simulink model "Full_Model_D_R5"  (R2013a)
settings: Solver=ode45  StartTime=0.0  StopTime=sim_length  MaxStep=1e-4  RelTol=1e-3
values from neighbouring files (symbols this model uses):
  A_Height_d = [1  0.03  0.00658443308606; 0  1  0.409781323477; 0  0  0.651439057531]    [Height_Controller_SS_D_Data.mat]    (also in Height_Controller_SS_D_Data[Conflict].mat; Height_Controller_Sample_Time.m = A_d; State_Space_Height_D_1.m = A_d)
  A_Roll_d = [1  0.03  0.0205960284122; 0  1  1.28179110803; 0  0  0.651439057531]    [Roll_Controller_SS_D_Data.mat]    (also in Roll_Controller_SS_D_Data[Conflict].mat; Roll_Controller_Sample_Time.m = A_d; State_Space_Roll_D_1.m = A_d)
  A_Yaw_d = A_d    [State_Space_Yaw_D_2.m]    (also in Yaw_Controller_SS_D_Data.mat = [1  0.03  0.0015367929619; 0  1  0.0956421070134; 0  0  0.65; Yaw_Controller_SS_D_Data[Conflict].mat = [1  0.03  0.0015367929619; 0  1  0.0956421070134; 0  0  0.65)
  B = [0 ... (first row only)    [Height_Controller_Sample_Time.m]    (also in Roll_Controller_Sample_Time.m; State_Space_Height_D_1.m; State_Space_Roll_D_1.m; State_Space_Yaw_D_2.m)
  B_Height_d = [0.000973236713115 0.0940633298008 0.348560942469]    [Height_Controller_SS_D_Data.mat]    (also in Height_Controller_SS_D_Data[Conflict].mat; Height_Controller_Sample_Time.m = B_d; State_Space_Height_D_1.m = B_d)
  B_Roll_d = [0.00304427286801 0.294228977317 0.348560942469]    [Roll_Controller_SS_D_Data.mat]    (also in Roll_Controller_SS_D_Data[Conflict].mat; Roll_Controller_Sample_Time.m = B_d; State_Space_Roll_D_1.m = B_d)
  B_Yaw_d = B_d    [State_Space_Yaw_D_2.m]    (also in Yaw_Controller_SS_D_Data.mat = [0.000231505127222 0.0222444322616 0.348560942469]; Yaw_Controller_SS_D_Data[Conflict].mat = [0.000231505127222 0.0222444322616 0.348560942469])
  C_Height_d = [1 0 0]    [Height_Controller_SS_D_Data.mat]    (also in Height_Controller_SS_D_Data[Conflict].mat; Height_Controller_Sample_Time.m = C_d; State_Space_Height_D_1.m = C_d)
  C_Roll_d = [1  0  0; 0  1  0]    [Roll_Controller_SS_D_Data.mat]    (also in Roll_Controller_SS_D_Data[Conflict].mat; Roll_Controller_Sample_Time.m = C_d; State_Space_Roll_D_1.m = C_d)
  C_Yaw_d = C_d    [State_Space_Yaw_D_2.m]    (also in Yaw_Controller_SS_D_Data.mat = [1  0  0; 0  1  0]; Yaw_Controller_SS_D_Data[Conflict].mat = [1  0  0; 0  1  0])
  Drag = D    [State_Space_Yaw_D_2.m]
  Feed_Forward_Height_d = 2    [Height_Controller_SS_D_Data.mat]    (also in Height_Controller_SS_D_Data[Conflict].mat; Height_Controller_Sample_Time.m; State_Space_Height_D_1.m)
  Feed_Forward_Roll_d = 1/8    (= 0.125)    [Height_Controller_Sample_Time.m]    (also in Roll_Controller_SS_D_Data.mat; Roll_Controller_SS_D_Data[Conflict].mat; Roll_Controller_Sample_Time.m; State_Space_Height_D_1.m)
  Feed_Forward_Yaw_d = 0    [State_Space_Yaw_D_2.m]    (also in Yaw_Controller_SS_D_Data.mat; Yaw_Controller_SS_D_Data[Conflict].mat)
  G_Height_d = [2.06012242861 38.4669769186 9.37529528927]    [Height_Controller_SS_D_Data.mat]    (also in Height_Controller_SS_D_Data[Conflict].mat; Height_Controller_Sample_Time.m = place(A_d',C_d',P)'; State_Space_Height_D_1.m = place(A_d',C_d',P)')
  G_Roll_d = [0.73387095133  0.036221570993; -0.0712605684884  1.12257105862; -0.0212805421137  0.11676537131]    [Roll_Controller_SS_D_Data.mat]    (also in Roll_Controller_SS_D_Data[Conflict].mat = [0.497083466726  0.0324399525972; -0.127651874026  0.6516223; Roll_Controller_Sample_Time.m = place(A_d',C_d',P)'; State_Space_Roll_D_1.m = place(A_d',C_d',P)')
  G_Yaw_d = place(A_d',C_d',P)'    [State_Space_Yaw_D_2.m]    (also in Yaw_Controller_SS_D_Data.mat = [0.190505534668  0.0274512375294; -0.00549182791178  0.03271; Yaw_Controller_SS_D_Data[Conflict].mat = [0.190505534668  0.0274512375294; -0.00549182791178  0.03271)
  K_Height_d = [2.39793427169 0.655884252958 0.592611157411]    [Height_Controller_SS_D_Data.mat]    (also in Height_Controller_SS_D_Data[Conflict].mat; Height_Controller_Sample_Time.m = K_Height_Reg(1:end-1); State_Space_Height_D_1.m = K_Height_Reg(1:end-1))
  K_Height_i = -1.9521886856    [Height_Controller_SS_D_Data.mat]    (also in Height_Controller_SS_D_Data[Conflict].mat; Height_Controller_Sample_Time.m = K_Height_Reg(end); State_Space_Height_D_1.m = K_Height_Reg(end))
  K_Roll_d = [1.02676834214 0.239868892992 0.659032552261]    [Roll_Controller_SS_D_Data.mat]    (also in Roll_Controller_SS_D_Data[Conflict].mat = [1.62241539227 0.326086850397 0.838371786069]; Roll_Controller_Sample_Time.m = K_Roll_Reg(1:end-1); State_Space_Roll_D_1.m = K_Roll_Reg(1:end-1))
  K_Roll_i = -1.92048833324    [Roll_Controller_SS_D_Data.mat]    (also in Roll_Controller_SS_D_Data[Conflict].mat = -1.83467215461; Roll_Controller_Sample_Time.m = K_Roll_Reg(end); State_Space_Roll_D_1.m = K_Roll_Reg(end))
  K_Yaw_d = K_Yaw_Reg(1:end-1)    [State_Space_Yaw_D_2.m]    (also in Yaw_Controller_SS_D_Data.mat = [0.370800639069 0.451703010874 0.117046660637]; Yaw_Controller_SS_D_Data[Conflict].mat = [0.370800639069 0.451703010874 0.117046660637])
  K_Yaw_i = K_Yaw_Reg(end)    [State_Space_Yaw_D_2.m]    (also in Yaw_Controller_SS_D_Data.mat = -0.131449182588; Yaw_Controller_SS_D_Data[Conflict].mat = -0.131449182588)
  NoiseMean = 0    [All_Controller_Sample_Time.m]
  omega_0 = 520    [State_Space_Yaw_D_2.m]    (also in Test_Controller_Sample_Time.m = (0-F_yIntercept)/Kf)
  omega_Lim = (0-F_yIntercept)/Kf    [Test_Controller_Sample_Time.m]
  Phi_IC = (0/180)*pi    (= 0)    [Test_Controller_Sample_Time.m]
  Pitch_Setpoint = 0    [Test_Controller_Sample_Time.m]
  PropDelay = 45e-3    (= 0.045)    [All_Controller_Sample_Time.m]
  Psi_IC = (0/180)*pi    (= 0)    [Test_Controller_Sample_Time.m]
  PWM_LimHigher = 2    [Test_Controller_Sample_Time.m]
  PWM_LimLower = 1.1    [Test_Controller_Sample_Time.m]
  Theta_IC = (5/180)*pi    (= 0.0872664625997)    [Test_Controller_Sample_Time.m]
  Ts = 30e-3    (= 0.03)    [All_Controller_Sample_Time.m]    (also in State_Space_Height_D_1.m = 0.02; State_Space_Roll_D_1.m = 0.02; State_Space_Yaw_D_2.m = 0.02)
  Yaw_Setpoint = 0    [Test_Controller_Sample_Time.m]
undefined symbols (not defined in the file or in its folder): DiscIntNeverNeededParam, F_yIntercept, g, I_Phi, I_Psi, I_Theta, J, Kf, Kw, L, Mass, Motor_TimeConstant, Speed_yIntercept
libraries: commnoisgen2 x7, simulink x6
settings Model: Creator=Ross  LastModifiedBy=Ross

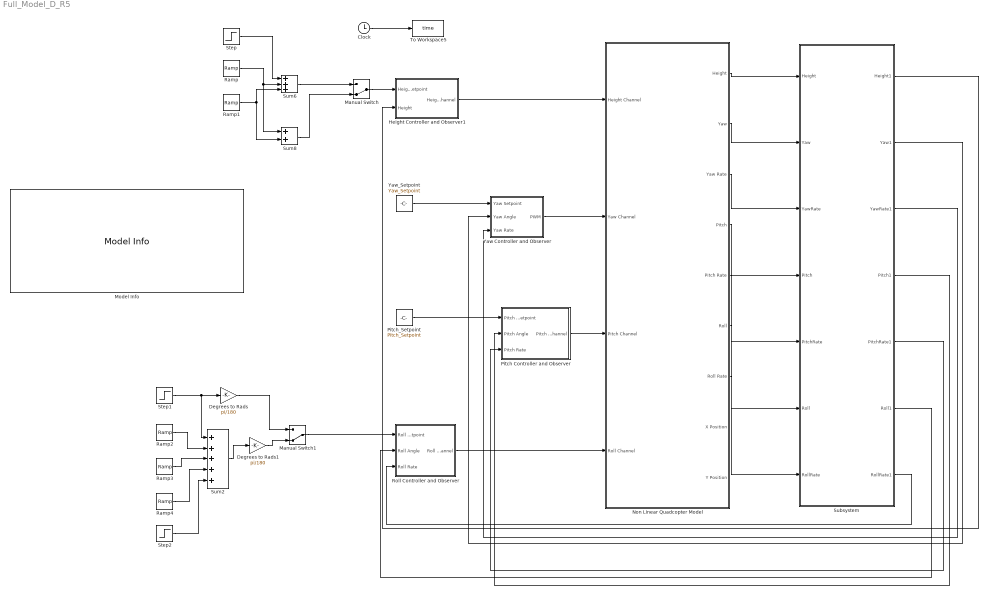
== system Full_Model_D_R5 ==
  Clock : Clock
  Degrees to Rads : Gain  Gain=pi/180
  Degrees to Rads1 : Gain  Gain=pi/180
  Height Controller and Observer1 : Subsystem
  Manual Switch : ManualSwitch  CurrentSetting=0
  Manual Switch1 : ManualSwitch  CurrentSetting=0
  Model Info : simulink/Model-Wide Utilities/Model Info  InitialBlockCM=None  BlockCM=None  Frame=on  DisplayStringWithTags=|  HorizontalTextAlignment=Center  LeftAlignmentValue=0.5  SourceBlockDiagram=Full_Model_D_R5  TagMaxNumber=20
      | %<ModelName>
      | Simulink Diagram Used in Testing of Controllers designed for Quadcopters
      | Model version is %<ModelVersion>
      | 
      | %<Created>
      | %<ModifiedBy>
      | %<ModifiedDate>
      | %<ModifiedComment>
      | 
      | 
      | %<LastModifiedBy>
      | %<LastModificationDate>
      | %<Description>
  Non Linear Quadcopter Model : Subsystem
  Pitch Controller and Observer : Subsystem
  "Pitch_Setpoint " : Constant  Value=Pitch_Setpoint
  Ramp : simulink/Sources/Ramp  slope=1  start=2  X0=0
  Ramp1 : simulink/Sources/Ramp  slope=-1  start=5  X0=0
  Ramp2 : simulink/Sources/Ramp  slope=0  start=2  X0=Ts
  Ramp3 : simulink/Sources/Ramp  slope=0  start=4  X0=Ts
  Ramp4 : simulink/Sources/Ramp  slope=0  start=6  X0=Ts
  Roll Controller and Observer : Subsystem
  Step : Step  Time=10  SampleTime=0
  Step1 : Step  Time=2  After=20  SampleTime=Ts
  Step2 : Step  Time=4  After=-20  SampleTime=Ts
  Subsystem : Subsystem
  Sum2 : Sum  Inputs=+++++
  Sum6 : Sum  Inputs=+++
  Sum8 : Sum
  To Workspace5 : ToWorkspace  VariableName=time  SampleTime=Ts  SaveFormat=Timeseries
  Yaw Controller and Observer : Subsystem
  Yaw_Setpoint : Constant  Value=Yaw_Setpoint
  wires:
  Ramp/1 -> Sum8/1, Sum6/2
  Ramp1/1 -> Sum8/2, Sum6/3
  Step/1 -> Sum6/1
  Manual Switch/1 -> Height Controller and Observer1/1(Height Setpoint)
  Sum8/1 -> Manual Switch/2
  Sum6/1 -> Manual Switch/1
  Ramp2/1 -> Sum2/2
  Ramp3/1 -> Sum2/3
  Step1/1 -> Sum2/1, Degrees to Rads/1
  Sum2/1 -> Degrees to Rads1/1
  Degrees to Rads/1 -> Manual Switch1/1
  "Pitch_Setpoint "/1 -> Pitch Controller and Observer/1(Pitch Setpoint)
  Manual Switch1/1 -> Roll Controller and Observer/1(Roll Setpoint)
  Yaw_Setpoint/1 -> Yaw Controller and Observer/1(Yaw Setpoint)
  Pitch Controller and Observer/1(Pitch Channel) -> Non Linear Quadcopter Model/3(Pitch Channel)
  Yaw Controller and Observer/1(PWM) -> Non Linear Quadcopter Model/2(Yaw Channel)
  Height Controller and Observer1/1(Height Channel) -> Non Linear Quadcopter Model/1(Height Channel)
  Degrees to Rads1/1 -> Manual Switch1/2
  Step2/1 -> Sum2/5
  Ramp4/1 -> Sum2/4
  Roll Controller and Observer/1(Roll Channel) -> Non Linear Quadcopter Model/4(Roll Channel)
  Non Linear Quadcopter Model/1(Height) -> Subsystem/1(Height)
  Non Linear Quadcopter Model/2(Yaw) -> Subsystem/2(Yaw)
  Non Linear Quadcopter Model/3(Yaw Rate) -> Subsystem/3(YawRate)
  Non Linear Quadcopter Model/4(Pitch) -> Subsystem/4(Pitch)
  Non Linear Quadcopter Model/5(Pitch Rate) -> Subsystem/5(PitchRate)
  Non Linear Quadcopter Model/6(Roll) -> Subsystem/6(Roll)
  Non Linear Quadcopter Model/7(Roll Rate) -> Subsystem/7(RollRate)
  Subsystem/1(Height1) -> Height Controller and Observer1/2(Height)
  Subsystem/2(Yaw1) -> Yaw Controller and Observer/2(Yaw Angle)
  Subsystem/3(YawRate1) -> Yaw Controller and Observer/3(Yaw Rate)
  Subsystem/4(Pitch1) -> Pitch Controller and Observer/2(Pitch Angle)
  Subsystem/5(PitchRate1) -> Pitch Controller and Observer/3(Pitch Rate)
  Subsystem/6("Roll1 ") -> Roll Controller and Observer/2(Roll Angle)
  Subsystem/7(RollRate1) -> Roll Controller and Observer/3(Roll Rate)
  Clock/1 -> To Workspace5/1

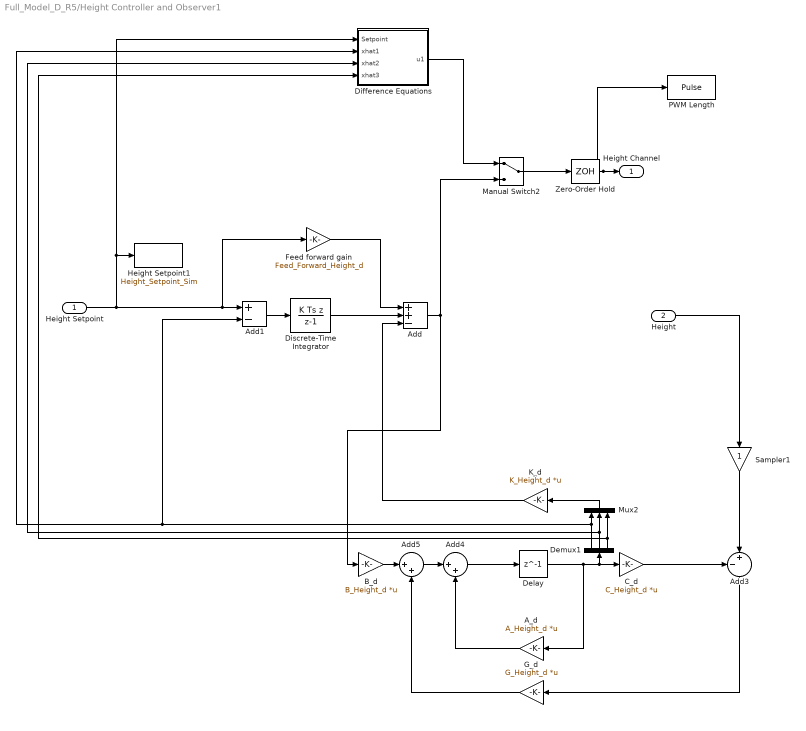
== system Full_Model_D_R5/Height Controller and Observer1 ==
  Height Setpoint : Inport
  Height : Inport  Port=2
  A_d : Gain  Gain=A_Height_d  Multiplication=Matrix(K*u)  SampleTime=Ts
  Add : Sum  Inputs=++-
  Add1 : Sum  Inputs=+-
  Add3 : Sum  Inputs=-+|
  Add4 : Sum  Inputs=|++
  Add5 : Sum  Inputs=|++
  "B_d " : Gain  Gain=B_Height_d  Multiplication=Matrix(K*u)  SampleTime=Ts
  "C_d " : Gain  Gain=C_Height_d  Multiplication=Matrix(K*u)  SampleTime=Ts
  Delay : Delay  DelayLength=1  InitialCondition=0  SampleTime=Ts
  Demux1 : Demux  Outputs=3
  Difference Equations : Subsystem
  Discrete-Time Integrator : DiscreteIntegrator  IntegratorMethod=Integration: Backward Euler  gainval=-K_Height_i  SampleTime=Ts  ICPrevOutput=DiscIntNeverNeededParam  ICPrevScaledInput=DiscIntNeverNeededParam
  Feed forward gain : Gain  Gain=Feed_Forward_Height_d  SampleTime=Ts
  G_d : Gain  Gain=G_Height_d  Multiplication=Matrix(K*u)  SampleTime=Ts
  Height Setpoint1 : ToWorkspace  VariableName=Height_Setpoint_Sim  SampleTime=-1  SaveFormat=Timeseries
  K_d : Gain  Gain=K_Height_d  Multiplication=Matrix(K*u)  SampleTime=Ts
  Manual Switch2 : ManualSwitch
  Mux2 : Mux  Inputs=3
  PWM Length : ToWorkspace  VariableName=Pulse  SampleTime=-1  SaveFormat=Timeseries
  Sampler1 : Gain  SampleTime=Ts
  Zero-Order Hold : ZeroOrderHold  SampleTime=Ts
  Height Channel : Outport
  wires:
  Add/1 -> Manual Switch2/2, "B_d "/1
  "B_d "/1 -> Add5/1
  K_d/1 -> Add/3
  Demux1/2 -> Difference Equations/3(xhat2), Mux2/2
  Sampler1/1 -> Add3/2
  Add4/1 -> Delay/1
  Add3/1 -> G_d/1
  Demux1/3 -> Mux2/3, Difference Equations/4(xhat3)
  Demux1/1 -> Difference Equations/2(xhat1), Add1/2, Mux2/1
  G_d/1 -> Add5/2
  Delay/1 -> Demux1/1, "C_d "/1, A_d/1
  Mux2/1 -> K_d/1
  "C_d "/1 -> Add3/1
  A_d/1 -> Add4/2
  Add5/1 -> Add4/1
  Height/1 -> Sampler1/1
  Height Setpoint/1 -> Difference Equations/1(Setpoint), Height Setpoint1/1, Feed forward gain/1, Add1/1
  Zero-Order Hold/1 -> PWM Length/1, Height Channel/1
  Feed forward gain/1 -> Add/1
  Add1/1 -> Discrete-Time Integrator/1
  Discrete-Time Integrator/1 -> Add/2
  Manual Switch2/1 -> Zero-Order Hold/1
  Difference Equations/1(u1) -> Manual Switch2/1

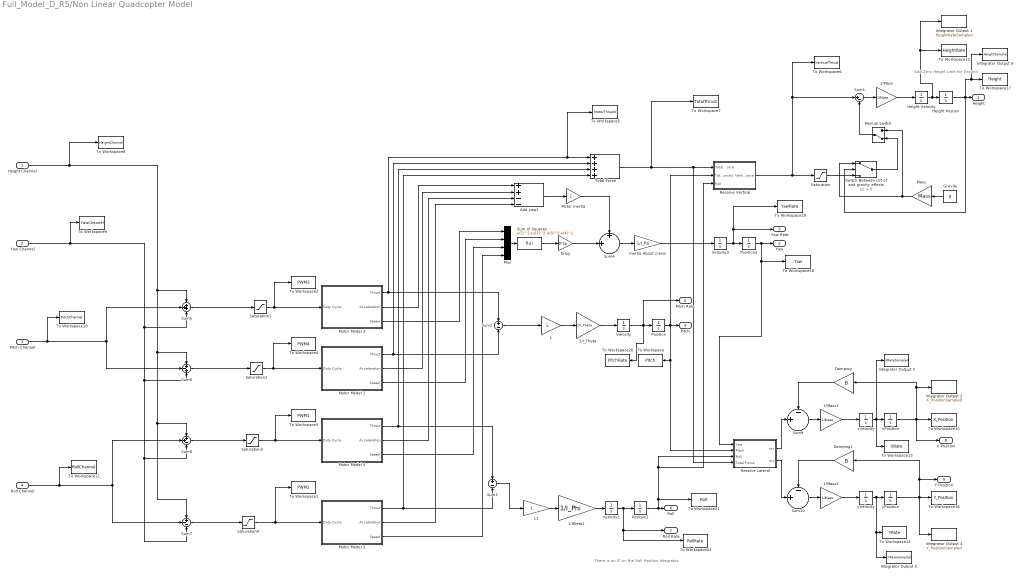
== system Full_Model_D_R5/Non Linear Quadcopter Model ==
  note: There is an IC on the Roll
      | Position Integrator
  note: Add Zero Height Limit
      | for Ground
  Height Channel : Inport
  Yaw Channel : Inport  Port=2
  Pitch Channel : Inport  Port=3
  Roll Channel : Inport  Port=4
  1/I_Theta : Gain  Gain=1/I_Theta
  1/Itheta1 : Gain  Gain=1/I_Phi
  1/Mass : Gain  Gain=1/Mass
  1/Mass1 : Gain  Gain=1/Mass
  1/Mass2 : Gain  Gain=1/Mass
  Add yaw1 : Sum  Inputs=++--
  Damping : Gain  Gain=B
  Damping1 : Gain  Gain=B
  Drag : Gain  Gain=Drag
  Gravity : Constant  Value=g
  Height Postion : Integrator  LowerSaturationLimit=0
  Height Velocity : Integrator
  Inertia About z-axis : Gain  Gain=1/I_Psi
  Integrator Output 1 : ToWorkspace  VariableName=HeightRateSampled  SampleTime=Ts  SaveFormat=Timeseries
  Integrator Output 2 : ToWorkspace  VariableName=X_PositionSampled  SampleTime=Ts  SaveFormat=Timeseries
  Integrator Output 3 : ToWorkspace  VariableName=XRateSampled  SampleTime=Ts  SaveFormat=Timeseries
  Integrator Output 4 : ToWorkspace  VariableName=Y_PositionSampled  SampleTime=Ts  SaveFormat=Timeseries
  Integrator Output 5 : ToWorkspace  VariableName=YRateSampled  SampleTime=Ts  SaveFormat=Timeseries
  Integrator Output 6 : ToWorkspace  VariableName=HeightSampled  SampleTime=Ts  SaveFormat=Timeseries
  L : Gain  Gain=L
  L1 : Gain  Gain=L
  Manual Switch : ManualSwitch  CurrentSetting=0
  Mass : Gain  Gain=Mass
  Motor Inertia : Gain  Gain=J
  Motor Model 1 : Subsystem
  Motor Model 2 : Subsystem
  Motor Model 3 : Subsystem
  Motor Model 4 : Subsystem
  Mux : Mux
  Position : Integrator  InitialCondition=Theta_IC
  Position1 : Integrator  InitialCondition=Phi_IC
  Position3 : Integrator  InitialCondition=Psi_IC
  Resolve Lateral : Subsystem
  Resolve Vertical : Subsystem
  Saturation : Saturate  UpperLimit=Mass*g  LowerLimit=-inf
  Saturation{1..4} (4 alike) : Saturate  UpperLimit=PWM_LimHigher  LowerLimit=PWM_LimLower
  Sum of Squares : Fcn  Expr=u(1)^2+u(2)^2-u(3)^2-u(4)^2
  Sum1 : Sum  Inputs=|+-
  Sum10 : Sum  Inputs=-|||+||||
  Sum2 : Sum  Inputs=+|-
  Sum3 : Sum  Inputs=+|-
  Sum4 : Sum  Inputs=+|||+||||
  Sum5 : Sum  Inputs=+++
  Sum6 : Sum  Inputs=+-+
  Sum7 : Sum  Inputs=+--
  Sum8 : Sum  Inputs=++-
  Sum9 : Sum  Inputs=-|||+||||
  Switch Between Lift of and gravity effects : Switch  Criteria=u2 > Threshold
  To Workspace : ToWorkspace  VariableName=Pitch  SampleTime=-1  SaveFormat=Timeseries
  To Workspace1 : ToWorkspace  VariableName=PWM2  SampleTime=-1  SaveFormat=Timeseries
  To Workspace10 : ToWorkspace  VariableName=PitchChannel  SampleTime=-1  SaveFormat=Timeseries
  To Workspace11 : ToWorkspace  VariableName=RollChannel  SampleTime=-1  SaveFormat=Timeseries
  To Workspace12 : ToWorkspace  VariableName=HeightRate  SampleTime=-1  SaveFormat=Timeseries
  To Workspace13 : ToWorkspace  VariableName=XRate  SampleTime=-1  SaveFormat=Timeseries
  To Workspace14 : ToWorkspace  VariableName=YRate  SampleTime=-1  SaveFormat=Timeseries
  To Workspace15 : ToWorkspace  VariableName=X_Position  SampleTime=-1  SaveFormat=Timeseries
  To Workspace16 : ToWorkspace  VariableName=Y_Position  SampleTime=-1  SaveFormat=Timeseries
  To Workspace17 : ToWorkspace  VariableName=Height  SampleTime=-1  SaveFormat=Timeseries
  To Workspace18 : ToWorkspace  VariableName=Yaw  SampleTime=-1  SaveFormat=Timeseries
  To Workspace19 : ToWorkspace  VariableName=YawRate  SampleTime=-1  SaveFormat=Timeseries
  To Workspace2 : ToWorkspace  VariableName=PWM3  SampleTime=-1  SaveFormat=Timeseries
  To Workspace20 : ToWorkspace  VariableName=PitchRate  SampleTime=-1  SaveFormat=Timeseries
  To Workspace21 : ToWorkspace  VariableName=Roll  SampleTime=-1  SaveFormat=Timeseries
  To Workspace22 : ToWorkspace  VariableName=RollRate  SampleTime=-1  SaveFormat=Timeseries
  To Workspace3 : ToWorkspace  VariableName=PWM1  SampleTime=-1  SaveFormat=Timeseries
  To Workspace4 : ToWorkspace  VariableName=PWM4  SampleTime=-1  SaveFormat=Timeseries
  To Workspace5 : ToWorkspace  VariableName=MotorThrust3  SampleTime=-1  SaveFormat=Timeseries
  To Workspace6 : ToWorkspace  VariableName=VerticalThrust  SampleTime=-1  SaveFormat=Timeseries
  To Workspace7 : ToWorkspace  VariableName=TotalThrust  SampleTime=-1  SaveFormat=Timeseries
  To Workspace8 : ToWorkspace  VariableName=HeightChannel  SampleTime=-1  SaveFormat=Timeseries
  To Workspace9 : ToWorkspace  VariableName=YawChannel  SampleTime=-1  SaveFormat=Timeseries
  Total Force : Sum  Inputs=++++
  Velocity : Integrator
  Velocity1 : Integrator
  Velocity3 : Integrator
  xPosition : Integrator
  xVelocity : Integrator
  yPosition : Integrator
  yVelocity : Integrator
  Height : Outport
  Yaw : Outport  Port=2
  Yaw Rate : Outport  Port=3
  Pitch : Outport  Port=4
  Pitch Rate : Outport  Port=5
  Roll : Outport  Port=6
  Roll Rate : Outport  Port=7
  X Position : Outport  Port=8
  Y Position : Outport  Port=9
  wires:
  Sum1/1 -> 1/Mass/1
  Pitch Channel/1 -> Sum6/2, Sum5/2, To Workspace10/1
  Add yaw1/1 -> Motor Inertia/1
  1/Mass/1 -> Height Velocity/1
  Motor Inertia/1 -> Sum4/1
  1/Mass1/1 -> xVelocity/1
  Sum9/1 -> 1/Mass1/1
  Damping/1 -> Sum9/1
  xVelocity/1 -> To Workspace13/1, Integrator Output 3/1, xPosition/1
  Motor Model 3/2(Acceleration) -> Add yaw1/1
  Sum8/1 -> Saturation3/1
  Sum2/1 -> L/1
  1/I_Theta/1 -> Velocity/1
  Velocity/1 -> To Workspace20/1, Pitch Rate/1, Position/1
  Position/1 -> Resolve Vertical/2(Total Force1), Pitch/1, To Workspace/1, Resolve Lateral/2(Pitch)
  Total Force/1 -> To Workspace7/1, Resolve Lateral/4(Total Force), Resolve Vertical/1(Total Force)
  Sum of Squares/1 -> Drag/1
  Drag/1 -> Sum4/2
  Position3/1 -> To Workspace18/1, Resolve Lateral/1(Yaw), Yaw/1
  Velocity3/1 -> To Workspace19/1, Yaw Rate/1, Position3/1
  Inertia About z-axis/1 -> Velocity3/1
  Motor Model 2/1(Thrust) -> Total Force/4, Sum3/2
  L1/1 -> 1/Itheta1/1
  Velocity1/1 -> To Workspace22/1, Roll Rate/1, Position1/1
  Sum3/1 -> L1/1
  Position1/1 -> Roll/1, To Workspace21/1, Resolve Lateral/3(Roll), Resolve Vertical/3(Roll)
  1/Itheta1/1 -> Velocity1/1
  Motor Model 3/1(Thrust) -> To Workspace5/1, Total Force/1, Sum2/1
  Sum10/1 -> 1/Mass2/1
  1/Mass2/1 -> yVelocity/1
  Damping1/1 -> Sum10/1
  yVelocity/1 -> Integrator Output 5/1, To Workspace14/1, yPosition/1
  Sum7/1 -> Saturation4/1
  Motor Model 4/2(Acceleration) -> Add yaw1/3
  Motor Model 1/1(Thrust) -> Total Force/2, Sum2/2
  Sum4/1 -> Inertia About z-axis/1
  Motor Model 4/1(Thrust) -> Total Force/3, Sum3/1
  Height Channel/1 -> To Workspace8/1, Sum6/1, Sum7/1, Sum8/1, Sum5/1
  Yaw Channel/1 -> To Workspace9/1, Sum7/3, Sum8/3, Sum6/3, Sum5/3
  Motor Model 1/2(Acceleration) -> Add yaw1/2
  Motor Model 2/2(Acceleration) -> Add yaw1/4
  Sum5/1 -> Saturation1/1
  Roll Channel/1 -> To Workspace11/1, Sum8/2, Sum7/2
  Gravity/1 -> Mass/1
  Resolve Lateral/1(mx) -> Sum9/2
  Resolve Lateral/2(my) -> Sum10/2
  Motor Model 3/3(Speed) -> Mux/1
  Motor Model 1/3(Speed) -> Mux/2
  Motor Model 4/3(Speed) -> Mux/3
  Motor Model 2/3(Speed) -> Mux/4
  Mux/1 -> Sum of Squares/1
  L/1 -> 1/I_Theta/1
  Switch Between Lift of and gravity effects/1 -> Manual Switch/2
  Saturation/1 -> Switch Between Lift of and gravity effects/3
  Mass/1 -> Manual Switch/1, Switch Between Lift of and gravity effects/1
  Sum6/1 -> Saturation2/1
  Manual Switch/1 -> Sum1/2
  Resolve Vertical/1(Vertical Force) -> Sum1/1, To Workspace6/1, Saturation/1
  yPosition/1 -> Y Position/1, Damping1/1, Integrator Output 4/1, To Workspace16/1
  Saturation1/1 -> Motor Model 3/1(Duty Cycle), To Workspace2/1
  Saturation2/1 -> Motor Model 1/1(Duty Cycle), To Workspace4/1
  Saturation3/1 -> Motor Model 4/1(Duty Cycle), To Workspace3/1
  Saturation4/1 -> Motor Model 2/1(Duty Cycle), To Workspace1/1
  Height Velocity/1 -> Integrator Output 1/1, To Workspace12/1, Height Postion/1
  xPosition/1 -> X Position/1, Damping/1, Integrator Output 2/1, To Workspace15/1
  Height Postion/1 -> Switch Between Lift of and gravity effects/2, Integrator Output 6/1, To Workspace17/1, Height/1

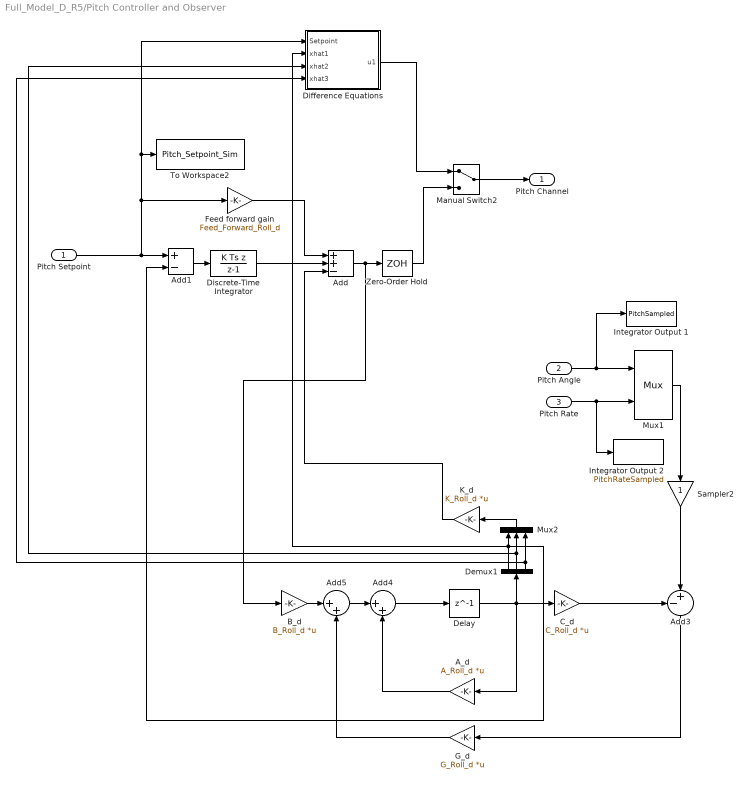
== system Full_Model_D_R5/Pitch Controller and Observer ==
  Pitch Setpoint : Inport
  Pitch Angle : Inport  Port=2
  Pitch Rate : Inport  Port=3
  A_d : Gain  Gain=A_Roll_d  Multiplication=Matrix(K*u)  SampleTime=Ts
  Add : Sum  Inputs=++-
  Add1 : Sum  Inputs=+-
  Add3 : Sum  Inputs=-+|
  Add4 : Sum  Inputs=|++
  Add5 : Sum  Inputs=|++
  "B_d " : Gain  Gain=B_Roll_d  Multiplication=Matrix(K*u)  SampleTime=Ts
  "C_d " : Gain  Gain=C_Roll_d  Multiplication=Matrix(K*u)  SampleTime=Ts
  Delay : Delay  DelayLength=1  InitialCondition=0  SampleTime=Ts
  Demux1 : Demux  Outputs=3
  Difference Equations : Subsystem
  Discrete-Time Integrator : DiscreteIntegrator  IntegratorMethod=Integration: Backward Euler  gainval=-K_Roll_i  SampleTime=Ts  ICPrevOutput=DiscIntNeverNeededParam  ICPrevScaledInput=DiscIntNeverNeededParam
  Feed forward gain : Gain  Gain=Feed_Forward_Roll_d  SampleTime=Ts
  G_d : Gain  Gain=G_Roll_d  Multiplication=Matrix(K*u)  SampleTime=Ts
  Integrator Output 1 : ToWorkspace  VariableName=PitchSampled  SampleTime=Ts  SaveFormat=Timeseries
  Integrator Output 2 : ToWorkspace  VariableName=PitchRateSampled  SampleTime=Ts  SaveFormat=Timeseries
  K_d : Gain  Gain=K_Roll_d  Multiplication=Matrix(K*u)  SampleTime=Ts
  Manual Switch2 : ManualSwitch
  Mux1 : Mux  Inputs=2
      settings: DisplayOption=signals
  Mux2 : Mux  Inputs=3
  Sampler2 : Gain  SampleTime=Ts
  To Workspace2 : ToWorkspace  VariableName=Pitch_Setpoint_Sim  SampleTime=-1  SaveFormat=Timeseries
  Zero-Order Hold : ZeroOrderHold  SampleTime=Ts
  Pitch Channel : Outport
  wires:
  Add5/1 -> Add4/1
  Demux1/3 -> Difference Equations/4(xhat3), Mux2/3
  Mux1/1 -> Sampler2/1
  G_d/1 -> Add5/2
  Demux1/2 -> Difference Equations/3(xhat2), Mux2/2
  A_d/1 -> Add4/2
  Add4/1 -> Delay/1
  "C_d "/1 -> Add3/1
  K_d/1 -> Add/3
  Sampler2/1 -> Add3/2
  Add/1 -> "B_d "/1, Zero-Order Hold/1
  "B_d "/1 -> Add5/1
  Mux2/1 -> K_d/1
  Add3/1 -> G_d/1
  Delay/1 -> "C_d "/1, Demux1/1, A_d/1
  Zero-Order Hold/1 -> Manual Switch2/2
  Discrete-Time Integrator/1 -> Add/2
  Pitch Setpoint/1 -> To Workspace2/1, Difference Equations/1(Setpoint), Feed forward gain/1, Add1/1
  Add1/1 -> Discrete-Time Integrator/1
  Feed forward gain/1 -> Add/1
  Pitch Angle/1 -> Integrator Output 1/1, Mux1/1
  Pitch Rate/1 -> Integrator Output 2/1, Mux1/2
  Difference Equations/1(u1) -> Manual Switch2/1
  Manual Switch2/1 -> Pitch Channel/1
  Demux1/1 -> Difference Equations/2(xhat1), Add1/2, Mux2/1

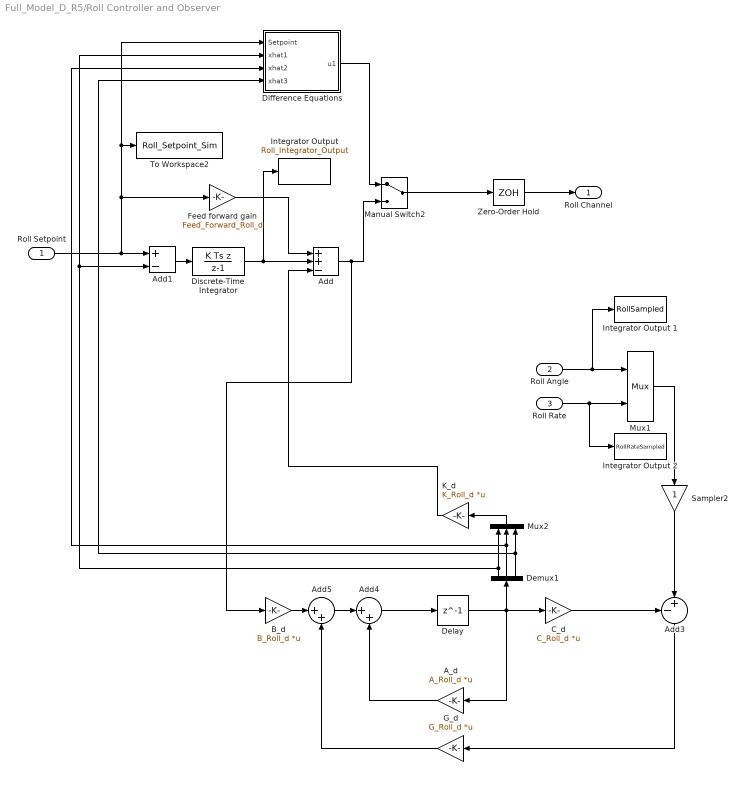
== system Full_Model_D_R5/Roll Controller and Observer ==
  Roll Setpoint : Inport
  Roll Angle : Inport  Port=2
  Roll Rate : Inport  Port=3
  A_d : Gain  Gain=A_Roll_d  Multiplication=Matrix(K*u)  SampleTime=Ts
  Add : Sum  Inputs=++-
  Add1 : Sum  Inputs=+-  SampleTime=Ts
  Add3 : Sum  Inputs=-+|
  Add4 : Sum  Inputs=|++
  Add5 : Sum  Inputs=|++
  "B_d " : Gain  Gain=B_Roll_d  Multiplication=Matrix(K*u)  SampleTime=Ts
  "C_d " : Gain  Gain=C_Roll_d  Multiplication=Matrix(K*u)  SampleTime=Ts
  Delay : Delay  DelayLength=1  InitialCondition=0  SampleTime=Ts
  Demux1 : Demux  Outputs=3
  Difference Equations : Subsystem
  Discrete-Time Integrator : DiscreteIntegrator  IntegratorMethod=Integration: Backward Euler  gainval=-K_Roll_i  SampleTime=Ts  ICPrevOutput=DiscIntNeverNeededParam  ICPrevScaledInput=DiscIntNeverNeededParam
  Feed forward gain : Gain  Gain=Feed_Forward_Roll_d  SampleTime=Ts
  G_d : Gain  Gain=G_Roll_d  Multiplication=Matrix(K*u)  SampleTime=Ts
  "Integrator Output " : ToWorkspace  VariableName=Roll_Integrator_Output  SampleTime=-1  SaveFormat=Timeseries
  Integrator Output 1 : ToWorkspace  VariableName=RollSampled  SampleTime=Ts  SaveFormat=Timeseries
  Integrator Output 2 : ToWorkspace  VariableName=RollRateSampled  SampleTime=Ts  SaveFormat=Timeseries
  K_d : Gain  Gain=K_Roll_d  Multiplication=Matrix(K*u)  SampleTime=Ts
  Manual Switch2 : ManualSwitch
  Mux1 : Mux  Inputs=2
      settings: DisplayOption=signals
  Mux2 : Mux  Inputs=3
  Sampler2 : Gain  SampleTime=Ts
  To Workspace2 : ToWorkspace  VariableName=Roll_Setpoint_Sim  SampleTime=-1  SaveFormat=Timeseries
  Zero-Order Hold : ZeroOrderHold  SampleTime=Ts
  Roll Channel : Outport
  wires:
  Add5/1 -> Add4/1
  Demux1/3 -> Difference Equations/4(xhat3), Mux2/3
  Mux1/1 -> Sampler2/1
  G_d/1 -> Add5/2
  A_d/1 -> Add4/2
  Add4/1 -> Delay/1
  "C_d "/1 -> Add3/1
  K_d/1 -> Add/3
  Sampler2/1 -> Add3/2
  "B_d "/1 -> Add5/1
  Mux2/1 -> K_d/1
  Add3/1 -> G_d/1
  Delay/1 -> "C_d "/1, Demux1/1, A_d/1
  Add/1 -> "B_d "/1, Manual Switch2/2
  Discrete-Time Integrator/1 -> "Integrator Output "/1, Add/2
  Add1/1 -> Discrete-Time Integrator/1
  Feed forward gain/1 -> Add/1
  Demux1/2 -> Mux2/2, Difference Equations/3(xhat2)
  Demux1/1 -> Difference Equations/2(xhat1), Add1/2, Mux2/1
  Roll Setpoint/1 -> Difference Equations/1(Setpoint), To Workspace2/1, Feed forward gain/1, Add1/1
  Manual Switch2/1 -> Zero-Order Hold/1
  Difference Equations/1(u1) -> Manual Switch2/1
  Zero-Order Hold/1 -> Roll Channel/1
  Roll Angle/1 -> Integrator Output 1/1, Mux1/1
  Roll Rate/1 -> Integrator Output 2/1, Mux1/2

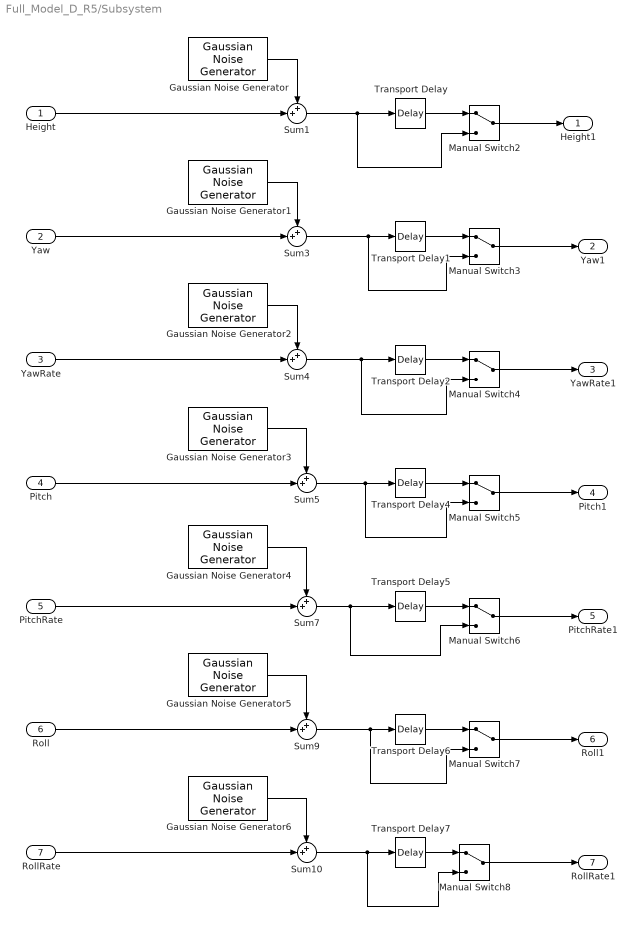
== system Full_Model_D_R5/Subsystem ==
  Height : Inport
  Yaw : Inport  Port=2
  YawRate : Inport  Port=3
  Pitch : Inport  Port=4
  PitchRate : Inport  Port=5
  Roll : Inport  Port=6
  RollRate : Inport  Port=7
  Gaussian Noise Generator : commnoisgen2/Gaussian Noise Generator  m=NoiseMean  d=NoiseHeightVariance  s=41  Ts=1  frameBased=off  sampPerFrame=1  orient=off  outDataType=double
  Gaussian Noise Generator1 : commnoisgen2/Gaussian Noise Generator  m=NoiseMean  d=NoiseAngleVariance  s=41  Ts=1  frameBased=off  sampPerFrame=1  orient=off  outDataType=double
  Gaussian Noise Generator2 : commnoisgen2/Gaussian Noise Generator  m=NoiseMean  d=NoiseAngleRateVariance  s=41  Ts=1  frameBased=off  sampPerFrame=1  orient=off  outDataType=double
  Gaussian Noise Generator3 : commnoisgen2/Gaussian Noise Generator  m=NoiseMean  d=NoiseAngleVariance  s=41  Ts=1  frameBased=off  sampPerFrame=1  orient=off  outDataType=double
  Gaussian Noise Generator4 : commnoisgen2/Gaussian Noise Generator  m=NoiseMean  d=NoiseAngleRateVariance  s=41  Ts=1  frameBased=off  sampPerFrame=1  orient=off  outDataType=double
  Gaussian Noise Generator5 : commnoisgen2/Gaussian Noise Generator  m=NoiseMean  d=NoiseAngleVariance  s=41  Ts=1  frameBased=off  sampPerFrame=1  orient=off  outDataType=double
  Gaussian Noise Generator6 : commnoisgen2/Gaussian Noise Generator  m=NoiseMean  d=NoiseAngleRateVariance  s=41  Ts=1  frameBased=off  sampPerFrame=1  orient=off  outDataType=double
  Manual Switch{2..8} (7 alike) : ManualSwitch
  Sum{1,3..5,7,9..10} (7 alike) : Sum  Inputs=++|
  Transport Delay{,1..2,4..7} (7 alike) : TransportDelay  DelayTime=PropDelay
  Height1 : Outport
  Yaw1 : Outport  Port=2
  YawRate1 : Outport  Port=3
  Pitch1 : Outport  Port=4
  PitchRate1 : Outport  Port=5
  "Roll1 " : Outport  Port=6
  RollRate1 : Outport  Port=7
  wires:
  Sum1/1 -> Manual Switch2/2, Transport Delay/1
  Transport Delay7/1 -> Manual Switch8/1
  Sum3/1 -> Manual Switch3/2, Transport Delay1/1
  Transport Delay2/1 -> Manual Switch4/1
  Transport Delay/1 -> Manual Switch2/1
  Transport Delay5/1 -> Manual Switch6/1
  Manual Switch2/1 -> Height1/1
  Sum7/1 -> Manual Switch6/2, Transport Delay5/1
  Transport Delay6/1 -> Manual Switch7/1
  Transport Delay4/1 -> Manual Switch5/1
  Gaussian Noise Generator2/1 -> Sum4/1
  Sum5/1 -> Manual Switch5/2, Transport Delay4/1
  Roll/1 -> Sum9/2
  Gaussian Noise Generator3/1 -> Sum5/1
  Gaussian Noise Generator/1 -> Sum1/1
  Sum10/1 -> Manual Switch8/2, Transport Delay7/1
  Gaussian Noise Generator4/1 -> Sum7/1
  Sum9/1 -> Manual Switch7/2, Transport Delay6/1
  Gaussian Noise Generator1/1 -> Sum3/1
  PitchRate/1 -> Sum7/2
  Gaussian Noise Generator6/1 -> Sum10/1
  Height/1 -> Sum1/2
  Yaw/1 -> Sum3/2
  RollRate/1 -> Sum10/2
  Pitch/1 -> Sum5/2
  Sum4/1 -> Manual Switch4/2, Transport Delay2/1
  Transport Delay1/1 -> Manual Switch3/1
  YawRate/1 -> Sum4/2
  Gaussian Noise Generator5/1 -> Sum9/1
  Manual Switch3/1 -> Yaw1/1
  Manual Switch8/1 -> RollRate1/1
  Manual Switch7/1 -> "Roll1 "/1
  Manual Switch6/1 -> PitchRate1/1
  Manual Switch5/1 -> Pitch1/1
  Manual Switch4/1 -> YawRate1/1

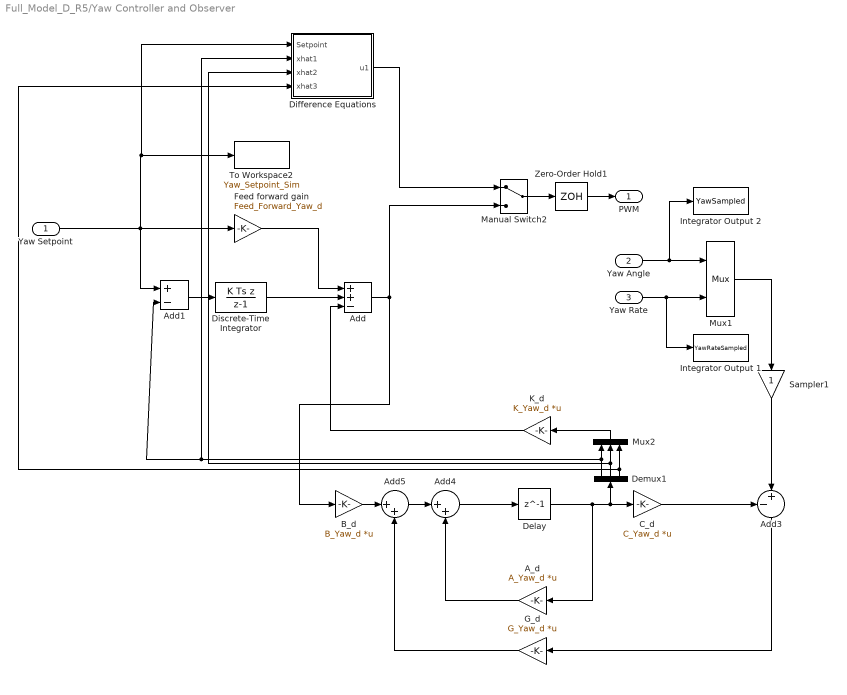
== system Full_Model_D_R5/Yaw Controller and Observer ==
  Yaw Setpoint : Inport
  Yaw Angle : Inport  Port=2
  Yaw Rate : Inport  Port=3
  A_d : Gain  Gain=A_Yaw_d  Multiplication=Matrix(K*u)  SampleTime=Ts
  Add : Sum  Inputs=++-
  Add1 : Sum  Inputs=+-
  Add3 : Sum  Inputs=-+|
  Add4 : Sum  Inputs=|++
  Add5 : Sum  Inputs=|++
  "B_d " : Gain  Gain=B_Yaw_d  Multiplication=Matrix(K*u)  SampleTime=Ts
  "C_d " : Gain  Gain=C_Yaw_d  Multiplication=Matrix(K*u)  SampleTime=Ts
  Delay : Delay  DelayLength=1  InitialCondition=0  SampleTime=Ts
  Demux1 : Demux  Outputs=3
  Difference Equations : Subsystem
  Discrete-Time Integrator : DiscreteIntegrator  IntegratorMethod=Integration: Backward Euler  gainval=-K_Yaw_i  SampleTime=Ts  ICPrevOutput=DiscIntNeverNeededParam  ICPrevScaledInput=DiscIntNeverNeededParam
  Feed forward gain : Gain  Gain=Feed_Forward_Yaw_d  SampleTime=Ts
  G_d : Gain  Gain=G_Yaw_d  Multiplication=Matrix(K*u)  SampleTime=Ts
  Integrator Output 1 : ToWorkspace  VariableName=YawRateSampled  SampleTime=Ts  SaveFormat=Timeseries
  Integrator Output 2 : ToWorkspace  VariableName=YawSampled  SampleTime=Ts  SaveFormat=Timeseries
  K_d : Gain  Gain=K_Yaw_d  Multiplication=Matrix(K*u)  SampleTime=Ts
  Manual Switch2 : ManualSwitch
  Mux1 : Mux  Inputs=2
      settings: DisplayOption=signals
  Mux2 : Mux  Inputs=3
  Sampler1 : Gain  SampleTime=Ts
  To Workspace2 : ToWorkspace  VariableName=Yaw_Setpoint_Sim  SampleTime=-1  SaveFormat=Timeseries
  Zero-Order Hold1 : ZeroOrderHold  SampleTime=Ts
  PWM : Outport
  wires:
  Yaw Setpoint/1 -> Add1/1, Difference Equations/1(Setpoint), To Workspace2/1, Feed forward gain/1
  Yaw Angle/1 -> Integrator Output 2/1, Mux1/1
  Yaw Rate/1 -> Integrator Output 1/1, Mux1/2
  Add1/1 -> Discrete-Time Integrator/1
  Demux1/1 -> Difference Equations/2(xhat1), Add1/2, Mux2/1
  Discrete-Time Integrator/1 -> Add/2
  Feed forward gain/1 -> Add/1
  Add/1 -> Manual Switch2/2, "B_d "/1
  Add3/1 -> G_d/1
  G_d/1 -> Add5/2
  Mux2/1 -> K_d/1
  Add5/1 -> Add4/1
  A_d/1 -> Add4/2
  Mux1/1 -> Sampler1/1
  Delay/1 -> Demux1/1, "C_d "/1, A_d/1
  Demux1/2 -> Mux2/2, Difference Equations/3(xhat2)
  Demux1/3 -> Difference Equations/4(xhat3), Mux2/3
  "B_d "/1 -> Add5/1
  "C_d "/1 -> Add3/1
  K_d/1 -> Add/3
  Add4/1 -> Delay/1
  Sampler1/1 -> Add3/2
  Difference Equations/1(u1) -> Manual Switch2/1
  Manual Switch2/1 -> Zero-Order Hold1/1
  Zero-Order Hold1/1 -> PWM/1

== system Full_Model_D_R5/Height Controller and Observer1/Difference Equations ==
  Setpoint : Inport
  xhat1 : Inport  Port=2
  xhat2 : Inport  Port=3
  xhat3 : Inport  Port=4
  Delay1 : Delay  DelayLength=1
  Mux : Mux  Inputs=5
  Mux3 : Mux  Inputs=3
  Roll Integator : Fcn  Expr=u(1) + ( -K_Height_i*Ts*( u(2)-u(3) ))  SampleTime=Ts
  Roll Regulator : Fcn  Expr=Feed_Forward_Height_d*u(1)+u(2)-K_Height_d(1)*u(3)-K_Height_d(2)*u(4)-K_Height_d(3)*u(5)  SampleTime=Ts
  u1 : Outport
  wires:
  Delay1/1 -> Mux3/1
  Mux/1 -> Roll Regulator/1
  xhat2/1 -> Mux/4
  xhat3/1 -> Mux/5
  xhat1/1 -> Mux/3, Mux3/3
  Setpoint/1 -> Mux3/2, Mux/1
  Roll Regulator/1 -> u1/1
  Roll Integator/1 -> Delay1/1, Mux/2  "v(k)"
  Mux3/1 -> Roll Integator/1

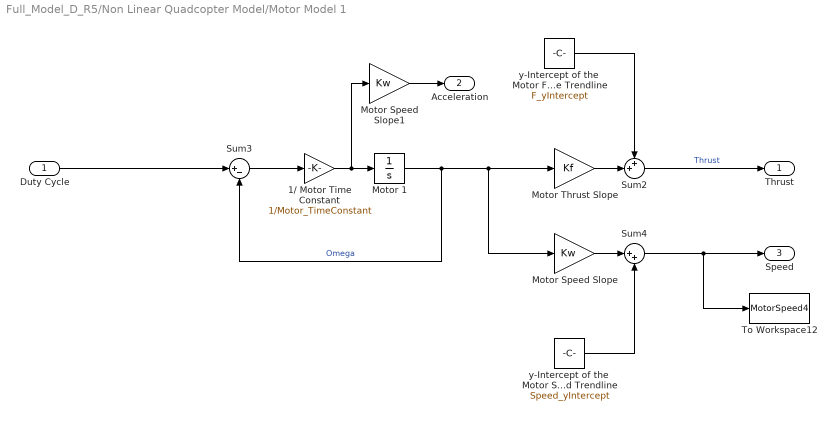
== system Full_Model_D_R5/Non Linear Quadcopter Model/Motor Model 1 ==
  Duty Cycle : Inport
  1/ Motor Time Constant : Gain  Gain=1/Motor_TimeConstant
  Motor 1 : Integrator  InitialCondition=omega_0  LimitOutput=on  LowerSaturationLimit=omega_Lim
  Motor Speed Slope : Gain  Gain=Kw
  Motor Speed Slope1 : Gain  Gain=Kw
  Motor Thrust Slope : Gain  Gain=Kf
  Sum2 : Sum  Inputs=++|
  Sum3 : Sum  Inputs=|+-
  Sum4 : Sum  Inputs=|++
  To Workspace12 : ToWorkspace  VariableName=MotorSpeed4  SampleTime=-1  SaveFormat=Timeseries
  y-Intercept of the  Motor Force Trendline : Constant  Value=F_yIntercept
  y-Intercept of the  Motor Speed Trendline : Constant  Value=Speed_yIntercept
  Thrust : Outport
  Acceleration : Outport  Port=2
  Speed : Outport  Port=3
  wires:
  Motor Thrust Slope/1 -> Sum2/2
  Motor 1/1 -> Sum3/2, Motor Speed Slope/1, Motor Thrust Slope/1  "Omega"
  Duty Cycle/1 -> Sum3/1
  Sum3/1 -> 1/ Motor Time Constant/1
  1/ Motor Time Constant/1 -> Motor 1/1, Motor Speed Slope1/1
  Motor Speed Slope/1 -> Sum4/1
  Motor Speed Slope1/1 -> Acceleration/1
  Sum2/1 -> Thrust/1  "Thrust"
  y-Intercept of the  Motor Force Trendline/1 -> Sum2/1
  y-Intercept of the  Motor Speed Trendline/1 -> Sum4/2
  Sum4/1 -> To Workspace12/1, Speed/1

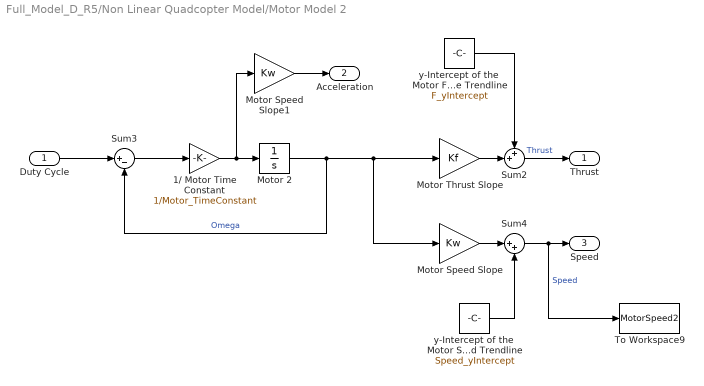
== system Full_Model_D_R5/Non Linear Quadcopter Model/Motor Model 2 ==
  Duty Cycle : Inport
  1/ Motor Time Constant : Gain  Gain=1/Motor_TimeConstant
  Motor 2 : Integrator  InitialCondition=omega_0  LimitOutput=on  LowerSaturationLimit=omega_Lim
  Motor Speed Slope : Gain  Gain=Kw
  Motor Speed Slope1 : Gain  Gain=Kw
  Motor Thrust Slope : Gain  Gain=Kf
  Sum2 : Sum  Inputs=++|
  Sum3 : Sum  Inputs=|+-
  Sum4 : Sum  Inputs=|++
  To Workspace9 : ToWorkspace  VariableName=MotorSpeed2  SampleTime=-1  SaveFormat=Timeseries
  y-Intercept of the  Motor Force Trendline : Constant  Value=F_yIntercept
  y-Intercept of the  Motor Speed Trendline : Constant  Value=Speed_yIntercept
  Thrust : Outport
  Acceleration : Outport  Port=2
  Speed : Outport  Port=3
  wires:
  Motor Thrust Slope/1 -> Sum2/2
  Motor 2/1 -> Sum3/2, Motor Speed Slope/1, Motor Thrust Slope/1  "Omega"
  Duty Cycle/1 -> Sum3/1
  Sum3/1 -> 1/ Motor Time Constant/1
  1/ Motor Time Constant/1 -> Motor 2/1, Motor Speed Slope1/1
  Motor Speed Slope/1 -> Sum4/1
  Motor Speed Slope1/1 -> Acceleration/1
  Sum2/1 -> Thrust/1  "Thrust"
  y-Intercept of the  Motor Force Trendline/1 -> Sum2/1
  Sum4/1 -> To Workspace9/1, Speed/1  "Speed"
  y-Intercept of the  Motor Speed Trendline/1 -> Sum4/2

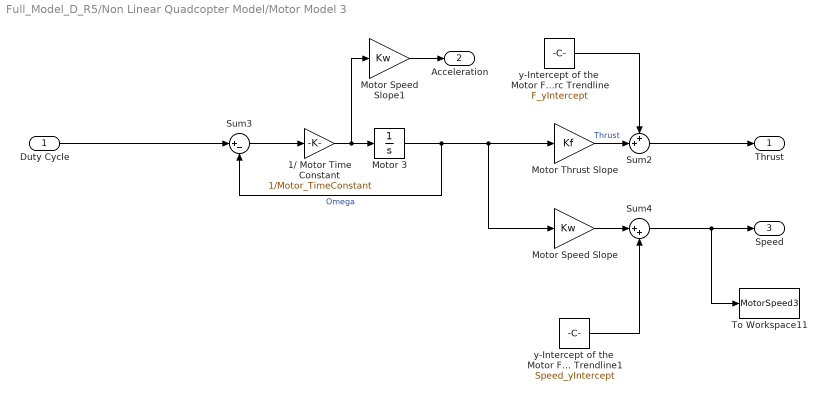
== system Full_Model_D_R5/Non Linear Quadcopter Model/Motor Model 3 ==
  Duty Cycle : Inport
  1/ Motor Time Constant : Gain  Gain=1/Motor_TimeConstant
  Motor 3 : Integrator  InitialCondition=omega_0  LimitOutput=on  LowerSaturationLimit=omega_Lim
  Motor Speed Slope : Gain  Gain=Kw
  Motor Speed Slope1 : Gain  Gain=Kw
  Motor Thrust Slope : Gain  Gain=Kf
  Sum2 : Sum  Inputs=++|
  Sum3 : Sum  Inputs=|+-
  Sum4 : Sum  Inputs=|++
  To Workspace11 : ToWorkspace  VariableName=MotorSpeed3  SampleTime=-1  SaveFormat=Timeseries
  y-Intercept of the  Motor Forc Trendline : Constant  Value=F_yIntercept
  y-Intercept of the  Motor Forc Trendline1 : Constant  Value=Speed_yIntercept
  Thrust : Outport
  Acceleration : Outport  Port=2
  Speed : Outport  Port=3
  wires:
  Motor Thrust Slope/1 -> Sum2/2  "Thrust"
  Motor 3/1 -> Sum3/2, Motor Speed Slope/1, Motor Thrust Slope/1  "Omega"
  Duty Cycle/1 -> Sum3/1
  Sum3/1 -> 1/ Motor Time Constant/1
  1/ Motor Time Constant/1 -> Motor 3/1, Motor Speed Slope1/1
  Motor Speed Slope/1 -> Sum4/1
  Motor Speed Slope1/1 -> Acceleration/1
  y-Intercept of the  Motor Forc Trendline/1 -> Sum2/1
  y-Intercept of the  Motor Forc Trendline1/1 -> Sum4/2
  Sum2/1 -> Thrust/1
  Sum4/1 -> To Workspace11/1, Speed/1

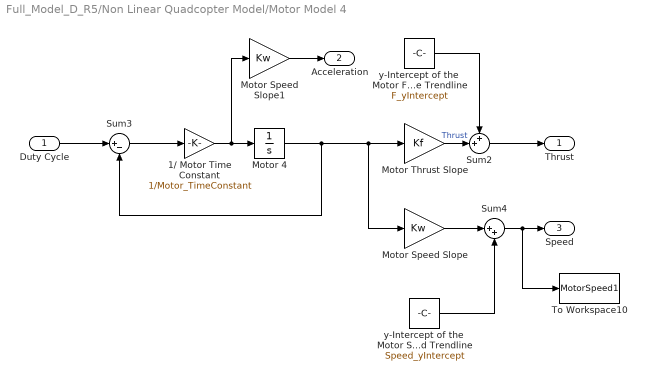
== system Full_Model_D_R5/Non Linear Quadcopter Model/Motor Model 4 ==
  Duty Cycle : Inport
  1/ Motor Time Constant : Gain  Gain=1/Motor_TimeConstant
  Motor 4 : Integrator  InitialCondition=omega_0  LimitOutput=on  LowerSaturationLimit=omega_Lim
  Motor Speed Slope : Gain  Gain=Kw
  Motor Speed Slope1 : Gain  Gain=Kw
  Motor Thrust Slope : Gain  Gain=Kf
  Sum2 : Sum  Inputs=++|
  Sum3 : Sum  Inputs=|+-
  Sum4 : Sum  Inputs=|++
  To Workspace10 : ToWorkspace  VariableName=MotorSpeed1  SampleTime=-1  SaveFormat=Timeseries
  y-Intercept of the  Motor Force Trendline : Constant  Value=F_yIntercept
  y-Intercept of the  Motor Speed Trendline : Constant  Value=Speed_yIntercept
  Thrust : Outport
  Acceleration : Outport  Port=2
  Speed : Outport  Port=3
  wires:
  Motor Thrust Slope/1 -> Sum2/2  "Thrust"
  Motor 4/1 -> Sum3/2, Motor Speed Slope/1, Motor Thrust Slope/1
  Duty Cycle/1 -> Sum3/1
  Sum3/1 -> 1/ Motor Time Constant/1
  1/ Motor Time Constant/1 -> Motor 4/1, Motor Speed Slope1/1
  Motor Speed Slope/1 -> Sum4/1
  Motor Speed Slope1/1 -> Acceleration/1
  Sum2/1 -> Thrust/1
  y-Intercept of the  Motor Force Trendline/1 -> Sum2/1
  Sum4/1 -> To Workspace10/1, Speed/1
  y-Intercept of the  Motor Speed Trendline/1 -> Sum4/2

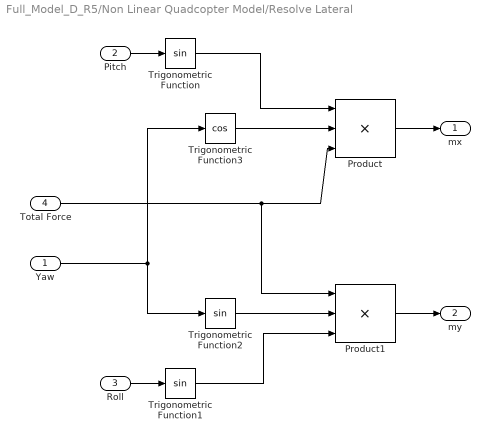
== system Full_Model_D_R5/Non Linear Quadcopter Model/Resolve Lateral ==
  Yaw : Inport
  Pitch : Inport  Port=2
  Roll : Inport  Port=3
  Total Force : Inport  Port=4
  Product : Product  Inputs=3
  Product1 : Product  Inputs=3
  Trigonometric Function : Trigonometry
  Trigonometric Function1 : Trigonometry
  Trigonometric Function2 : Trigonometry
  Trigonometric Function3 : Trigonometry  Operator=cos
  mx : Outport
  my : Outport  Port=2
  wires:
  Trigonometric Function/1 -> Product/1
  Total Force/1 -> Product1/1, Product/3
  Product/1 -> mx/1
  Roll/1 -> Trigonometric Function1/1
  Trigonometric Function1/1 -> Product1/3
  Product1/1 -> my/1
  Trigonometric Function3/1 -> Product/2
  Trigonometric Function2/1 -> Product1/2
  Yaw/1 -> Trigonometric Function2/1, Trigonometric Function3/1
  Pitch/1 -> Trigonometric Function/1

== system Full_Model_D_R5/Non Linear Quadcopter Model/Resolve Vertical ==
  Total Force : Inport
  Total Force1 : Inport  Port=2
  Roll : Inport  Port=3
  Product : Product  Inputs=3
  Trigonometric Function : Trigonometry  Operator=cos
  Trigonometric Function1 : Trigonometry  Operator=cos
  Vertical Force : Outport
  wires:
  Trigonometric Function/1 -> Product/1
  Total Force/1 -> Product/3
  Roll/1 -> Trigonometric Function1/1
  Total Force1/1 -> Trigonometric Function/1
  Product/1 -> Vertical Force/1
  Trigonometric Function1/1 -> Product/2

== system Full_Model_D_R5/Pitch Controller and Observer/Difference Equations ==
  Setpoint : Inport
  xhat1 : Inport  Port=2
  xhat2 : Inport  Port=3
  xhat3 : Inport  Port=4
  Delay1 : Delay  DelayLength=1
  Mux : Mux  Inputs=5
  Mux3 : Mux  Inputs=3
  Roll Integator : Fcn  Expr=u(1) + ( -K_Roll_i*Ts*( u(2)-u(3) ))  SampleTime=Ts
  Roll Regulator : Fcn  Expr=Feed_Forward_Roll_d*u(1)+u(2)-K_Roll_d(1)*u(3)-K_Roll_d(2)*u(4)-K_Roll_d(3)*u(5)  SampleTime=Ts
  u1 : Outport
  wires:
  Delay1/1 -> Mux3/1
  Mux/1 -> Roll Regulator/1
  xhat2/1 -> Mux/4
  xhat3/1 -> Mux/5
  xhat1/1 -> Mux/3, Mux3/3
  Setpoint/1 -> Mux3/2, Mux/1
  Roll Regulator/1 -> u1/1
  Roll Integator/1 -> Delay1/1, Mux/2  "v(k)"
  Mux3/1 -> Roll Integator/1

== system Full_Model_D_R5/Roll Controller and Observer/Difference Equations ==
  Setpoint : Inport
  xhat1 : Inport  Port=2
  xhat2 : Inport  Port=3
  xhat3 : Inport  Port=4
  Delay1 : Delay  DelayLength=1
  Mux : Mux  Inputs=5
  Mux3 : Mux  Inputs=3
  Roll Integator : Fcn  Expr=u(1) + ( -K_Roll_i*Ts*( u(2)-u(3) ))  SampleTime=Ts
  Roll Regulator : Fcn  Expr=Feed_Forward_Roll_d*u(1)+u(2)-K_Roll_d(1)*u(3)-K_Roll_d(2)*u(4)-K_Roll_d(3)*u(5)  SampleTime=Ts
  u1 : Outport
  wires:
  Delay1/1 -> Mux3/1
  Mux/1 -> Roll Regulator/1
  xhat2/1 -> Mux/4
  xhat3/1 -> Mux/5
  xhat1/1 -> Mux/3, Mux3/3
  Setpoint/1 -> Mux3/2, Mux/1
  Roll Regulator/1 -> u1/1
  Roll Integator/1 -> Delay1/1, Mux/2  "v(k)"
  Mux3/1 -> Roll Integator/1

== system Full_Model_D_R5/Yaw Controller and Observer/Difference Equations ==
  Setpoint : Inport
  xhat1 : Inport  Port=2
  xhat2 : Inport  Port=3
  xhat3 : Inport  Port=4
  Delay1 : Delay  DelayLength=1
  Mux : Mux  Inputs=5
  Mux3 : Mux  Inputs=3
  Roll Integator : Fcn  Expr=u(1) + ( -K_Yaw_i*Ts*( u(2)-u(3) ))  SampleTime=Ts
  Roll Regulator : Fcn  Expr=Feed_Forward_Yaw_d*u(1)+u(2)-K_Yaw_d(1)*u(3)-K_Yaw_d(2)*u(4)-K_Yaw_d(3)*u(5)  SampleTime=Ts
  u1 : Outport
  wires:
  Delay1/1 -> Mux3/1
  Mux/1 -> Roll Regulator/1
  xhat2/1 -> Mux/4
  xhat3/1 -> Mux/5
  xhat1/1 -> Mux/3, Mux3/3
  Setpoint/1 -> Mux3/2, Mux/1
  Roll Regulator/1 -> u1/1
  Roll Integator/1 -> Delay1/1, Mux/2  "v(k)"
  Mux3/1 -> Roll Integator/1
